simulink model "SchemSimulink"  (R2022a)
settings: Solver=VariableStepAuto  StartTime=0.0  StopTime=1.2  RelTol=1e-3
values from neighbouring files (symbols this model uses):
  Gzas = tf([1],conv([1 -0.2],[1 -0.1]),Tc)    [es7.m]
  Tc = 0.001    [Esercizio10_controllore.m]    (also in es7.m = 0.01)
undefined symbols (not defined in the file or in its folder): C3
settings Model: Creator=chiar  LastModifiedBy=Stefano
settings SolverCC: AlgebraicLoopSolver=TrustRegion
settings DebuggingCC: UnconnectedInputMsg=warning  UnconnectedOutputMsg=warning  UnconnectedLineMsg=warning  SFMachineParentedDataDiag=warning
settings RTWCC: DLArmComputeVersion=19.05

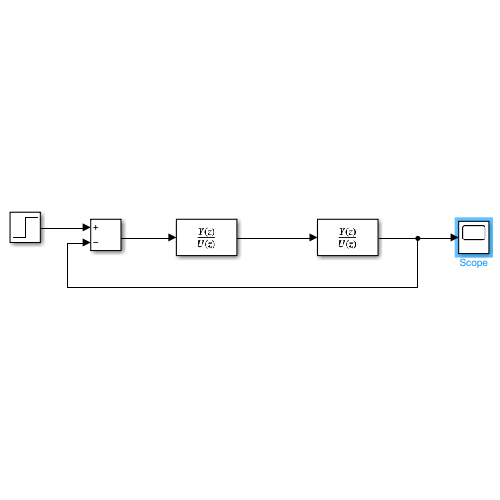
[thumbnail: Simulink's stored preview of the top-level diagram]
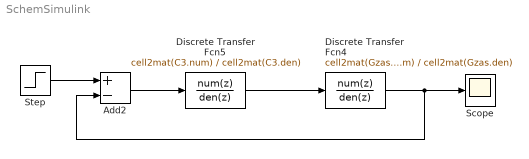
== system SchemSimulink ==
  Add2 : Sum  Inputs=+-
  Discrete Transfer Fcn4 : DiscreteTransferFcn  Numerator=cell2mat(Gzas.num)  Denominator=cell2mat(Gzas.den)  SampleTime=Tc
  Discrete Transfer Fcn5 : DiscreteTransferFcn  Numerator=cell2mat(C3.num)  Denominator=cell2mat(C3.den)  SampleTime=Tc
  Scope : Scope
  Step : Step  SampleTime=0
  wires:
  Step/1 -> Add2/1
  Discrete Transfer Fcn4/1 -> Scope/1, Add2/2
  Discrete Transfer Fcn5/1 -> Discrete Transfer Fcn4/1
  Add2/1 -> Discrete Transfer Fcn5/1
